simulink model "lab2"  (R2022b)
settings: Solver=VariableStepAuto  StartTime=0.0  StopTime=10.0  RelTol=1e-3
undefined symbols (not defined in the file or in its folder): K
libraries: simulink x1
settings Model: Creator=fwah  LastModifiedBy=fwah

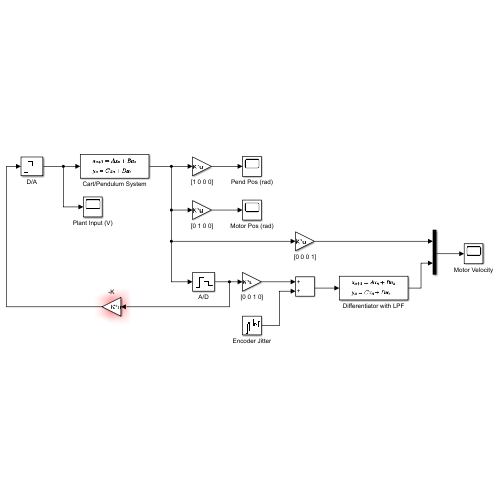
[thumbnail: Simulink's stored preview of the top-level diagram]
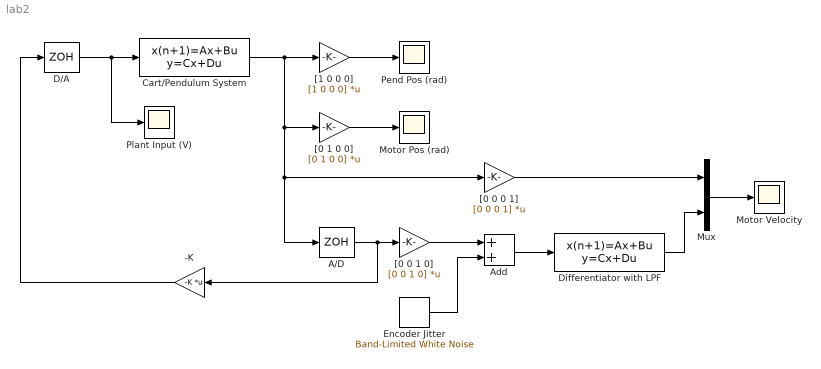
== system lab2 ==
  -K : Gain  Gain=-K  Multiplication=Matrix(K*u)
  A/D : ZeroOrderHold  SampleTime=-1
  Add : Sum
  Cart/Pendulum System : DiscreteStateSpace  SampleTime=-1
  D/A : ZeroOrderHold  SampleTime=-1
  Differentiator with LPF : DiscreteStateSpace  SampleTime=-1
  Encoder Jitter : simulink/Sources/Band-Limited White Noise  Cov=[0.1]  Ts=0.1  seed=[23341]
  Motor Pos (rad) : Scope
  Motor Velocity : Scope
  Mux : Mux  Inputs=2
  Pend Pos (rad) : Scope
  Plant Input (V) : Scope
  "[0 0 0 1]" : Gain  Gain=[0 0 0 1]  Multiplication=Matrix(K*u)
  "[0 0 1 0]" : Gain  Gain=[0 0 1 0]  Multiplication=Matrix(K*u)
  "[0 1 0 0]" : Gain  Gain=[0 1 0 0]  Multiplication=Matrix(K*u)
  "[1 0 0 0]" : Gain  Gain=[1 0 0 0]  Multiplication=Matrix(K*u)
  wires:
  Encoder Jitter/1 -> Add/2
  A/D/1 -> -K/1, "[0 0 1 0]"/1
  -K/1 -> D/A/1
  D/A/1 -> Plant Input (V)/1, Cart/Pendulum System/1
  "[0 0 1 0]"/1 -> Add/1
  Cart/Pendulum System/1 -> "[0 0 0 1]"/1, A/D/1, "[0 1 0 0]"/1, "[1 0 0 0]"/1
  "[0 1 0 0]"/1 -> Motor Pos (rad)/1
  "[1 0 0 0]"/1 -> Pend Pos (rad)/1
  "[0 0 0 1]"/1 -> Mux/1
  Add/1 -> Differentiator with LPF/1
  Differentiator with LPF/1 -> Mux/2
  Mux/1 -> Motor Velocity/1
